simulink library "Turbine_State_Machine_Lib"  (R2019b)
settings: Solver=ode45  StartTime=0.0  StopTime=10.0  RelTol=1e-3  EnableMultiTasking=on
Description:
  | Copyright 2009-2017 The MathWorks, Inc. MathWorks, Inc.
settings Model: Creator=smiller  LastModifiedBy=bhisma
settings DataIOCC: LimitDataPoints=on  SaveFormat=Array  SignalLoggingSaveFormat=ModelDataLogs  ReturnWorkspaceOutputs=off
settings OptimizationCC: ExpressionDepthLimit=2147483647  LifeSpan=inf
settings DebuggingCC: UnderspecifiedInitializationDetection=Classic  MergeDetectMultiDrivingBlocksExec=none  SolverPrmCheckMsg=warning  FcnCallInpInsideContextMsg=warning  AllowSymbolicDim=off  StateNameClashWarn=warning  SFUnexpectedBacktrackingDiag=warning  SFNoUnconditionalDefaultTransitionDiag=warning  SFExecutionAtInitializationDiag=none  ArithmeticOperatorsInVariantConditions=warning
settings HardwareCC: ProdBitPerPointer=32  ProdBitPerSizeT=32  ProdBitPerPtrDiffT=32  ProdLargestAtomicFloat=None  ProdIntDivRoundTo=Undefined  ProdEndianess=Unspecified  ProdWordSize=32  ProdHWDeviceType=32-bit Generic
settings ModelReferenceCC: PropagateSignalLabelsOutOfModel=off
settings SFSimCC: SimUseLocalCustomCode=off  CustomCodeUndefinedFunction=UseInterfaceOnly
settings RTWCC: RTWUseLocalCustomCode=off
settings CodeAppCC: StateflowObjectComments=on
settings GRTTargetCC: TargetLangStandard=C89/C90 (ANSI)  GeneratePreprocessorConditionals=Disable all  CombineOutputUpdateFcns=off  GRTInterface=on
settings ConfigComp: CovMetricSettings=dw  CovHtmlReporting=on  CovSaveCumulativeToWorkspaceVar=on  CovSaveSingleToWorkspaceVar=on  CovExternalEMLEnable=off  CovSFcnEnable=off

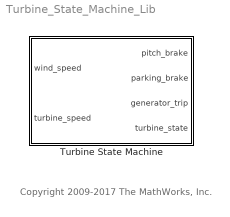
== system Turbine_State_Machine_Lib ==
  note: Copyright 2009-2017 The MathWorks, Inc.
  Turbine State Machine : Stateflow chart  TreatAsAtomicUnit=on

== stateflow chart Turbine_State_Machine_Lib/Turbine State Machine ==
  state Generating
    entry: parking_brake = 0;
    generator_trip = 0;
    pitch_brake = 0;
    turbine_state = 2;
  state Startup
    entry: parking_brake = 0;
    generator_trip = 1;
    pitch_brake = 0;
    turbine_state = 1;
  state Park
    entry: parking_brake = 1;
    generator_trip = 1;
    pitch_brake = 1;
    turbine_state = 0;
  state Brake
    entry: parking_brake = 0;
    generator_trip = 1;
    pitch_brake = 1;
    turbine_state = 3;
  Startup -> Generating [order 1] : [turbine_speed>...
      | turbine_speed_cut_in]
  Park -> Startup : [wind_speed>...
      | wind_speed_cut_in_lower...
      | &&wind_speed<...
      | wind_speed_cut_out]
  Startup -> Brake [order 2] : [wind_speed<...
      | wind_speed_cut_in_lower]
  Brake -> Startup [order 2] : [wind_speed<...
      | wind_speed_cut_in_upper...
      | && wind_speed>...
      | wind_speed_cut_in_lower]
  Generating -> Brake : [wind_speed<...
      | wind_speed_cut_in_lower...
      | ||wind_speed>...
      | wind_speed_cut_out...
      | ||turbine_speed>...
      | turbine_speed_cut_out...
      | ||turbine_speed<...
      | turbine_speed_cut_in*0.9]
  (default) -> Park
  Brake -> Park [order 1] : [turbine_speed<=...
      | park_speed]
  data: pitch_brake output double; wind_speed input; turbine_speed input; parking_brake output double; generator_trip output double; wind_speed_cut_in_lower local double =WT_Params.Main_Controller.wind_speed_cut_in_lower; turbine_speed_cut_in local double =WT_Params.Main_Controller.turbine_speed_cut_in; turbine_state output double; wind_speed_cut_out local double =WT_Params.Main_Controller.wind_speed_cut_out; wind_speed_cut_in_upper local double =WT_Params.Main_Controller.wind_speed_cut_in_upper; turbine_speed_cut_out local double =WT_Params.Main_Controller.turbine_speed_cut_out; park_speed constant double =WT_Params.Main_Controller.turbine_speed_park
